simulink model "digital_filter"  (Simulink 6.2)
settings: Solver=ode45  StartTime=0.0  StopTime=1  RelTol=1e-3
libraries: dspsrcs4 x2, dspsigops x2, dsparch4 x1
settings Model: LastModifiedBy=PHYSICS
settings DebuggingCC: SolverPrmCheckMsg=warning

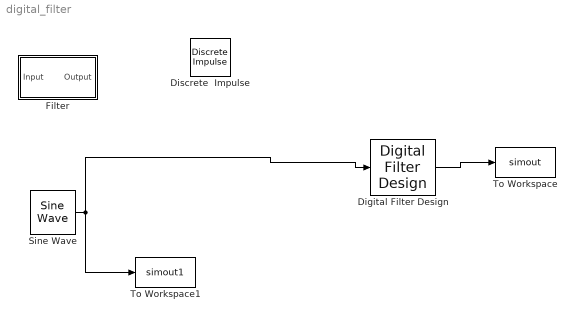
== system digital_filter ==
  Digital Filter Design : dsparch4/Digital Filter Design  mwdsp_browser_bugfix_var=off
  Discrete  Impulse : dspsrcs4/Discrete  Impulse  Delay=0  SampleTime=1/20000  FrameSample=1  dataType=double  isSigned=on  wordLen=16  udDataType=sfix(16)  fracBitsMode=Best precision  numFracBits=15
  Filter : Subsystem  Tag=FilterWizardSubSystem
      settings: ErrorFcn=dspFilterRealizedInBasicElemsAlgLoopErrFcnCallback
  Sine Wave : dspsrcs4/Sine Wave  Amplitude=1  Frequency=10  Phase=0  SampleMode=Discrete  OutComplex=Real  CompMethod=Trigonometric fcn  TableSize=Speed  SampleTime=1/20000  SamplesPerFrame=1  dataType=double  wordLen=16  udDataType=sfix(16)  fracBitsMode=Best precision  numFracBits=15  ResetState=Restart at time zero
  To Workspace : ToWorkspace  VariableName=simout  SampleTime=-1  SaveFormat=Array
  To Workspace1 : ToWorkspace  VariableName=simout1  SampleTime=-1  SaveFormat=Array
  wires:
  Sine Wave/1 -> Digital Filter Design/1, To Workspace1/1
  Digital Filter Design/1 -> To Workspace/1

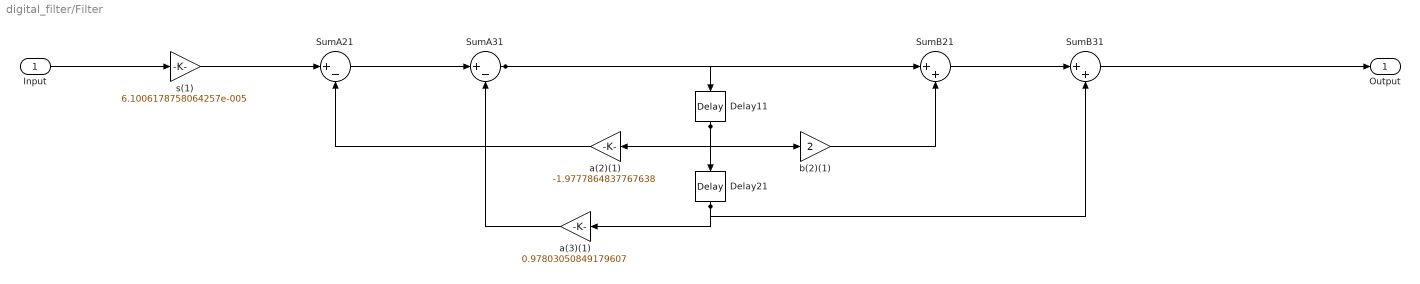
== system digital_filter/Filter ==
  Input : Inport  Port=1  LatchInput=off
  Delay11 : dspsigops/Delay  Orientation=down  dly_unit=Samples  delay=1  ic_detail=off  dif_ic_for_ch=off  dif_ic_for_dly=off  ic=0  reset_popup=None
  Delay21 : dspsigops/Delay  Orientation=down  dly_unit=Samples  delay=1  ic_detail=off  dif_ic_for_ch=off  dif_ic_for_dly=off  ic=0  reset_popup=None
  SumA21 : Sum  Inputs=|+-  SaturateOnIntegerOverflow=on  InputSameDT=on
  SumA31 : Sum  Inputs=|+-  SaturateOnIntegerOverflow=on  InputSameDT=on
  SumB21 : Sum  Inputs=|++  SaturateOnIntegerOverflow=on  InputSameDT=on
  SumB31 : Sum  Inputs=|++  SaturateOnIntegerOverflow=on  InputSameDT=on
  a(2)(1) : Gain  Orientation=left  Gain=-1.9777864837767638  SaturateOnIntegerOverflow=on
  a(3)(1) : Gain  Orientation=left  Gain=0.97803050849179607  SaturateOnIntegerOverflow=on
  b(2)(1) : Gain  Gain=2  SaturateOnIntegerOverflow=on
  s(1) : Gain  Gain=6.1006178758064257e-005  SaturateOnIntegerOverflow=on
  Output : Outport
  wires:
  Input/1 -> s(1)/1
  s(1)/1 -> SumA21/1
  SumA21/1 -> SumA31/1
  SumA31/1 -> SumB21/1, Delay11/1
  SumB21/1 -> SumB31/1
  SumB31/1 -> Output/1
  a(2)(1)/1 -> SumA21/2
  Delay11/1 -> a(2)(1)/1, b(2)(1)/1, Delay21/1
  b(2)(1)/1 -> SumB21/2
  a(3)(1)/1 -> SumA31/2
  Delay21/1 -> a(3)(1)/1, SumB31/2
